simulink model "Test3S150Board_HSMA"  (Simulink 6.4)
settings: Solver=ode45  SolverMode=SingleTasking  StartTime=0.0  StopTime=1000.0  FixedStep=1  RelTol=1e-3
InitFcn:
  | %% DSPBuilder Start
  | alt_dspbuilder_update_model(bdroot)
  | %% DSPBuilder End
undefined symbols (not defined in the file): Pin_AA1, Pin_AA6, Pin_AA7, Pin_AB1, Pin_AB10, Pin_AB2, Pin_AB3, Pin_AB5, Pin_AB6, Pin_AB8, Pin_AC1, Pin_AC11, Pin_AC2, Pin_AC4, Pin_AC5, Pin_AC6, Pin_AC7, Pin_AC8, Pin_AC9, Pin_AD1, Pin_AD6, Pin_AD7, Pin_AE1, Pin_AE2, Pin_AE3, Pin_AE4, Pin_AE7, Pin_AE8, Pin_AF1, Pin_AF2, Pin_AF5, Pin_AF6, Pin_AG3, Pin_AG4, Pin_AH2, Pin_AH4, Pin_AH5, Pin_AJ1, Pin_AJ2, Pin_AJ3, Pin_AJ4, Pin_AJ9, Pin_AK1, Pin_AK9, Pin_AL1, Pin_AL2, Pin_AL7, Pin_AL9, Pin_AM1, Pin_AM2, Pin_Y10, Pin_Y5, Pin_Y6, Pin_Y7, Pin_Y8, Pin_Y9
libraries: allblocks_alteradspbuilder2 x49, Stratix_III_EP3SL150_alteradspbuilder2 x5
settings Model: Creator=lkong  LastModifiedBy=lkong
settings DataIOCC: SignalLoggingName=sigsOut
settings OptimizationCC: InlineInvariantSignals=on
settings DebuggingCC: SolverPrmCheckMsg=none  StrictBusMsg=None
settings HardwareCC: TargetUnknown=on
settings GRTTargetCC: ModelReferenceCompliant=off  MatFileLogging=off

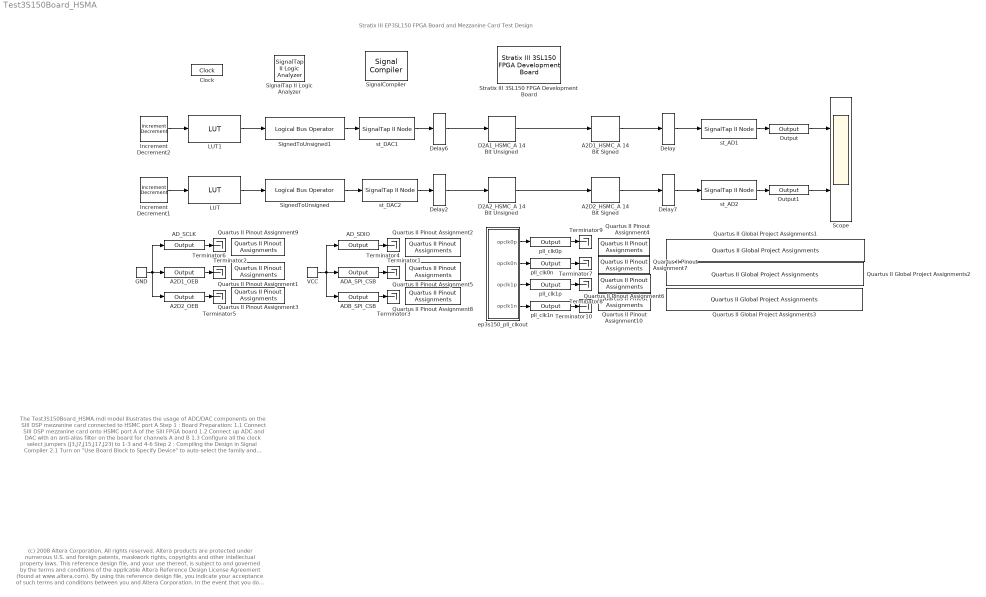
== system Test3S150Board_HSMA ==
  note: Stratix III EP3SL150 FPGA Board and Mezzanine Card Test Design
  note: (c) 2008 Altera Corporation. All rights reserved.  Altera products are protected under numerous U.S. and foreign patents, maskwork rights, copyrights and other intellectual property laws.
      | This reference design file, and your use thereof, is subject to and governed by the terms and conditions of the applicable Altera Reference Design License Agreement (found at www.altera.com).
      | By using this reference design file, you indicate your acceptance of such terms and conditions between you and Altera Corporation.
      | In the event that you do not agree with such terms and conditions, you may not use the reference design file and please promptly destroy any copies you have made.
      | This reference design file being provided on an "as-is" basis and as an accommodation and therefore all warranties, representations or guarantees of any kind (whether express, implied or statutory)
      | including, without limitation, warranties of merchantability, non-infringement, or fitness for a particular purpose, are specifically disclaimed.
      | By making this reference design file available, Altera expressly does not recommend, suggest or require that this reference design file be used in combination with any other product not provided by Altera
  note: The Test3S150Board_HSMA.mdl model illustrates the usage of ADC/DAC components on the SIII DSP mezzanine card connected to HSMC port A
      |
      | Step 1 : Board Preparation:
      |                1.1 Connect SIII DSP mezzanine card onto HSMC port A of the SIII FPGA board
      |                1.2 Connect up ADC and DAC with an anti-alias filter on the board for channels A and B
      |                1.3 Configure all the clock select jumpers (J3,J7,J15,J17,J23) to 1-3 and 4-6
      | Step 2 : Compiling the Design in Signal Compiler
      |                2.1 Turn on "Use Board Block to Specify Device" to auto-select the family and device
      |                2.2 Click "Compile" to compile the design through the Quartus II software and create a .sof file
      |                2.3 Click "Scan Jtag" to select a download cable and device
      |                2.4 Click "Program" to download the .sof file onto the FPGA device
      | Step 3 : Running SignalTap II Logic Analyzer
      |                3.1 Click "Scan Jtag" to select a download cable and device
      |                3.2 Click "Acquire" to obtain data for embedded SignalTap II nodes
  A2D1_HSMC_A 14 Bit Signed : Stratix_III_EP3SL150_alteradspbuilder2/A2D1_HSMC_A 14 Bit Signed  iofile=d:\ws80\workspace\Documentation\DesignExamples\Demos\Board\StratixIII_DSPBoard_3S150\tb_Test3S150Board_HSMA\Test3S150Board%5FHSMA_A2D1%5FHSMC%5FA+14+Bit+Signed.salt  externalType=Inferred  SpecifyClock=off  location=Pin_AD6,Pin_AD7,Pin_AF5,Pin_AF6,Pin_AE7,Pin_AE8,Pin_AH4,Pin_AH5,Pin_AC8,Pin_AC9,Pin_AB10,Pin_AC11,Pin_AL7,Pin_AK9
  A2D1_OEB : allblocks_alteradspbuilder2/Output  iofile=d:\ws80\workspace\Documentation\DesignExamples\Demos\Board\StratixIII_DSPBoard_3S150\tb_Test3S150Board_HSMA\Test3S150Board%5FHSMA_A2D1%5FOEB.capture  BusType=Single Bit  bwl=1  bwr=0  externalType=Inferred  PORTTYPE=Output  allowFloatingPointOverride=on  logOutputs=off
  A2D2_HSMC_A 14 Bit Signed : Stratix_III_EP3SL150_alteradspbuilder2/A2D2_HSMC_A 14 Bit Signed  iofile=d:\ws80\workspace\Documentation\DesignExamples\Demos\Board\StratixIII_DSPBoard_3S150\tb_Test3S150Board_HSMA\Test3S150Board%5FHSMA_A2D2%5FHSMC%5FA+14+Bit+Signed.salt  externalType=Inferred  SpecifyClock=off  location=Pin_AJ1,Pin_AH2,Pin_AK1,Pin_AJ2,Pin_AL1,Pin_AL2,Pin_AM1,Pin_AM2,Pin_AG3,Pin_AG4,Pin_AJ3,Pin_AJ4,Pin_AL9,Pin_AJ9
  A2D2_OEB : allblocks_alteradspbuilder2/Output  iofile=d:\ws80\workspace\Documentation\DesignExamples\Demos\Board\StratixIII_DSPBoard_3S150\tb_Test3S150Board_HSMA\Test3S150Board%5FHSMA_A2D2%5FOEB.capture  BusType=Single Bit  bwl=1  bwr=0  externalType=Inferred  PORTTYPE=Output  allowFloatingPointOverride=on  logOutputs=off
  ADA_SPI_CSB : allblocks_alteradspbuilder2/Output  iofile=d:\ws80\workspace\Documentation\DesignExamples\Demos\Board\StratixIII_DSPBoard_3S150\tb_Test3S150Board_HSMA\Test3S150Board%5FHSMA_ADA%5FSPI%5FCSB.capture  BusType=Single Bit  bwl=1  bwr=0  externalType=Inferred  PORTTYPE=Output  allowFloatingPointOverride=on  logOutputs=off
  ADB_SPI_CSB : allblocks_alteradspbuilder2/Output  iofile=d:\ws80\workspace\Documentation\DesignExamples\Demos\Board\StratixIII_DSPBoard_3S150\tb_Test3S150Board_HSMA\Test3S150Board%5FHSMA_ADB%5FSPI%5FCSB.capture  BusType=Single Bit  bwl=1  bwr=0  externalType=Inferred  PORTTYPE=Output  allowFloatingPointOverride=on  logOutputs=off
  AD_SCLK : allblocks_alteradspbuilder2/Output  iofile=d:\ws80\workspace\Documentation\DesignExamples\Demos\Board\StratixIII_DSPBoard_3S150\tb_Test3S150Board_HSMA\Test3S150Board%5FHSMA_AD%5FSCLK.capture  BusType=Single Bit  bwl=1  bwr=0  externalType=Inferred  PORTTYPE=Output  allowFloatingPointOverride=on  logOutputs=off
  AD_SDIO : allblocks_alteradspbuilder2/Output  iofile=d:\ws80\workspace\Documentation\DesignExamples\Demos\Board\StratixIII_DSPBoard_3S150\tb_Test3S150Board_HSMA\Test3S150Board%5FHSMA_AD%5FSDIO.capture  BusType=Single Bit  bwl=1  bwr=0  externalType=Inferred  PORTTYPE=Output  allowFloatingPointOverride=on  logOutputs=off
  Clock : allblocks_alteradspbuilder2/Clock  ClockPeriod=20  ClockPeriodUnit=ns  SampleTime=1  SimulationStartCycle=5  PhaseOffset=0  Reset=aclr  ResetType=Active Low  Export=off
  D2A1_HSMC_A 14 Bit Unsigned : Stratix_III_EP3SL150_alteradspbuilder2/D2A1_HSMC_A 14 Bit Unsigned  iofile=d:\ws80\workspace\Documentation\DesignExamples\Demos\Board\StratixIII_DSPBoard_3S150\tb_Test3S150Board_HSMA\Test3S150Board%5FHSMA_D2A1%5FHSMC%5FA+14+Bit+Unsigned.capture  externalType=Inferred  location=Pin_Y9,Pin_Y10,Pin_Y7,Pin_Y8,Pin_AA6,Pin_AA7,Pin_Y5,Pin_Y6,Pin_AC7,Pin_AB8,Pin_AB5,Pin_AB6,Pin_AC5,Pin_AC6
  D2A2_HSMC_A 14 Bit Unsigned : Stratix_III_EP3SL150_alteradspbuilder2/D2A2_HSMC_A 14 Bit Unsigned  iofile=d:\ws80\workspace\Documentation\DesignExamples\Demos\Board\StratixIII_DSPBoard_3S150\tb_Test3S150Board_HSMA\Test3S150Board%5FHSMA_D2A2%5FHSMC%5FA+14+Bit+Unsigned.capture  externalType=Inferred  location=Pin_AB3,Pin_AC4,Pin_AB1,Pin_AA1,Pin_AC1,Pin_AB2,Pin_AD1,Pin_AC2,Pin_AE3,Pin_AE4,Pin_AE1,Pin_AE2,Pin_AF1,Pin_AF2
  Delay : allblocks_alteradspbuilder2/Delay  pipeline=1  pipeline_display=1  ClockPhase=1  use_ena=off  use_sclr=off  allowFloatingPointOverride=on  logOutputs=off  logFile=d:\ws80\workspace\Documentation\DesignExamples\Demos\Board\StratixIII_DSPBoard_3S150\tb_Test3S150Board_HSMA\Test3S150Board%5FHSMA_Delay.fixedpointlog  use_init=off  reset_value=1
  Delay2 : allblocks_alteradspbuilder2/Delay  pipeline=1  pipeline_display=1  ClockPhase=1  use_ena=off  use_sclr=off  allowFloatingPointOverride=on  logOutputs=off  logFile=d:\ws80\workspace\Documentation\DesignExamples\Demos\Board\StratixIII_DSPBoard_3S150\tb_Test3S150Board_HSMA\Test3S150Board%5FHSMA_Delay2.fixedpointlog  use_init=off  reset_value=1
  Delay6 : allblocks_alteradspbuilder2/Delay  pipeline=1  pipeline_display=1  ClockPhase=1  use_ena=off  use_sclr=off  allowFloatingPointOverride=on  logOutputs=off  logFile=d:\ws80\workspace\Documentation\DesignExamples\Demos\Board\StratixIII_DSPBoard_3S150\tb_Test3S150Board_HSMA\Test3S150Board%5FHSMA_Delay6.fixedpointlog  use_init=off  reset_value=1
  Delay7 : allblocks_alteradspbuilder2/Delay  pipeline=1  pipeline_display=1  ClockPhase=1  use_ena=off  use_sclr=off  allowFloatingPointOverride=on  logOutputs=off  logFile=d:\ws80\workspace\Documentation\DesignExamples\Demos\Board\StratixIII_DSPBoard_3S150\tb_Test3S150Board_HSMA\Test3S150Board%5FHSMA_Delay7.fixedpointlog  use_init=off  reset_value=1
  GND : allblocks_alteradspbuilder2/GND  SpecifyClock=off
  Increment Decrement1 : allblocks_alteradspbuilder2/Increment Decrement  BusType=Unsigned Integer  bwl=7  bwr=0  SpecifyClock=off  clr_value=0  direction=Increment  phase_selection=1  use_ena=off  use_sclr=off  pipeline_display=1
  Increment Decrement2 : allblocks_alteradspbuilder2/Increment Decrement  BusType=Unsigned Integer  bwl=7  bwr=0  SpecifyClock=off  clr_value=0  direction=Increment  phase_selection=1  use_ena=off  use_sclr=off  pipeline_display=1
  LUT : allblocks_alteradspbuilder2/LUT  addr_width=7  BusType=Signed Integer  bwl=14  bwr=0  init_array=8191*sin( [0:2*pi/(2^7):2*pi] )  allowFloatingPointOverride=on  logOutputs=off  logFile=d:\ws80\workspace\Documentation\DesignExamples\Demos\Board\StratixIII_DSPBoard_3S150\tb_Test3S150Board_HSMA\Test3S150Board%5FHSMA_LUT.fixedpointlog  use_ena=off  reg_data=on  use_lpm=on  reg_addr=on  ram_type=AUTO  pipeline_display=2
  LUT1 : allblocks_alteradspbuilder2/LUT  addr_width=7  BusType=Signed Integer  bwl=14  bwr=0  init_array=8191*sin( [0:2*pi/(2^7):2*pi] )  allowFloatingPointOverride=on  logOutputs=off  logFile=d:\ws80\workspace\Documentation\DesignExamples\Demos\Board\StratixIII_DSPBoard_3S150\tb_Test3S150Board_HSMA\Test3S150Board%5FHSMA_LUT1.fixedpointlog  use_ena=off  reg_data=on  use_lpm=on  reg_addr=on  ram_type=AUTO  pipeline_display=2
  Output : allblocks_alteradspbuilder2/Output  iofile=d:\ws80\workspace\Documentation\DesignExamples\Demos\Board\StratixIII_DSPBoard_3S150\tb_Test3S150Board_HSMA\Test3S150Board%5FHSMA_Output.capture  BusType=Signed Integer  bwl=14  bwr=0  externalType=Inferred  PORTTYPE=Output  allowFloatingPointOverride=on  logOutputs=off
  Output1 : allblocks_alteradspbuilder2/Output  iofile=d:\ws80\workspace\Documentation\DesignExamples\Demos\Board\StratixIII_DSPBoard_3S150\tb_Test3S150Board_HSMA\Test3S150Board%5FHSMA_Output1.capture  BusType=Signed Integer  bwl=14  bwr=0  externalType=Inferred  PORTTYPE=Output  allowFloatingPointOverride=on  logOutputs=off
  Quartus II Global Project Assignments1 : allblocks_alteradspbuilder2/Quartus II Global Project Assignments  QuartusIIAssignmentName=RESERVE_DATA1_AFTER_CONFIGURATION  QuartusIIAssignmentValue="\"USE AS REGULAR IO\""
  Quartus II Global Project Assignments2 : allblocks_alteradspbuilder2/Quartus II Global Project Assignments  QuartusIIAssignmentName=RESERVE_NCEO_AFTER_CONFIGURATION  QuartusIIAssignmentValue="\"USE AS REGULAR IO\""
  Quartus II Global Project Assignments3 : allblocks_alteradspbuilder2/Quartus II Global Project Assignments  QuartusIIAssignmentName=RESERVE_DCLK_AFTER_CONFIGURATION  QuartusIIAssignmentValue="\"USE AS REGULAR IO\""
  Quartus II Pinout Assignment1 : allblocks_alteradspbuilder2/Quartus II Pinout Assignments  QuartusIIAssignmentName=A2D1_OEB  QuartusIIAssignmentValue=Pin_AE5
  Quartus II Pinout Assignment10 : allblocks_alteradspbuilder2/Quartus II Pinout Assignments  QuartusIIAssignmentName=pll_clk1n  QuartusIIAssignmentValue=Pin_W7
  Quartus II Pinout Assignment2 : allblocks_alteradspbuilder2/Quartus II Pinout Assignments  QuartusIIAssignmentName=AD_SDIO  QuartusIIAssignmentValue=Pin_AD3
  Quartus II Pinout Assignment3 : allblocks_alteradspbuilder2/Quartus II Pinout Assignments  QuartusIIAssignmentName=A2D2_OEB  QuartusIIAssignmentValue=Pin_AF3
  Quartus II Pinout Assignment4 : allblocks_alteradspbuilder2/Quartus II Pinout Assignments  QuartusIIAssignmentName=pll_clk0p  QuartusIIAssignmentValue=Pin_V10
  Quartus II Pinout Assignment5 : allblocks_alteradspbuilder2/Quartus II Pinout Assignments  QuartusIIAssignmentName=ADA_SPI_CSB  QuartusIIAssignmentValue=Pin_AD4
  Quartus II Pinout Assignment6 : allblocks_alteradspbuilder2/Quartus II Pinout Assignments  QuartusIIAssignmentName=pll_clk1p  QuartusIIAssignmentValue=Pin_W8
  Quartus II Pinout Assignment7 : allblocks_alteradspbuilder2/Quartus II Pinout Assignments  QuartusIIAssignmentName=pll_clk0n  QuartusIIAssignmentValue=Pin_W9
  Quartus II Pinout Assignment8 : allblocks_alteradspbuilder2/Quartus II Pinout Assignments  QuartusIIAssignmentName=ADB_SPI_CSB  QuartusIIAssignmentValue=Pin_AG1
  Quartus II Pinout Assignment9 : allblocks_alteradspbuilder2/Quartus II Pinout Assignments  QuartusIIAssignmentName=AD_SCLK  QuartusIIAssignmentValue=Pin_AH1
  Scope : Scope  NumInputPorts=2
      settings: YMin=-5~-5  YMax=5~5  SampleInput=on
  SignalCompiler : allblocks_alteradspbuilder2/Signal Compiler  DeviceFamily=Stratix III  DeviceName=EP3SL150F1152C4  EnableSignalTap=on  SignalTapDepth=512  UseBoardBlock=on  StpUseDefaultClock=on  StpClock=Clock  ExportDir=D:\MATLAB\R2006a\work
  SignalTap II Logic Analyzer : allblocks_alteradspbuilder2/SignalTap II Logic Analyzer
  SignedToUnsigned : allblocks_alteradspbuilder2/Logical Bus Operator  BusType=Unsigned Integer  bwl=14  bwr=0  LogicalOp_text=XOR  mask_value_num=8192  shift_amount=3  force_sign_ext=off  pipeline_display=0
  SignedToUnsigned1 : allblocks_alteradspbuilder2/Logical Bus Operator  BusType=Unsigned Integer  bwl=14  bwr=0  LogicalOp_text=XOR  mask_value_num=8192  shift_amount=3  force_sign_ext=off  pipeline_display=0
  "Stratix III 3SL150 FPGA Development Board " : Stratix_III_EP3SL150_alteradspbuilder2/Stratix III 3SL150 FPGA Development Board   ClockPinIn=Pin_T33  GlobalResetPin=PIN_AP5  device=EP3SL150F1152C4
  Terminator{1..10} (10 alike) : Terminator
  VCC : allblocks_alteradspbuilder2/VCC  SpecifyClock=off
  ep3s150_pll_clkout : Subsystem
      mask Type: SubSystem AlteraBlockSet
  pll_clk0n : allblocks_alteradspbuilder2/Output  iofile=d:\ws80\workspace\Documentation\DesignExamples\Demos\Board\StratixIII_DSPBoard_3S150\tb_Test3S150Board_HSMA\Test3S150Board%5FHSMA_pll%5Fclk0n.capture  BusType=Single Bit  bwl=1  bwr=0  externalType=Inferred  PORTTYPE=Output  allowFloatingPointOverride=on  logOutputs=off
  pll_clk0p : allblocks_alteradspbuilder2/Output  iofile=d:\ws80\workspace\Documentation\DesignExamples\Demos\Board\StratixIII_DSPBoard_3S150\tb_Test3S150Board_HSMA\Test3S150Board%5FHSMA_pll%5Fclk0p.capture  BusType=Single Bit  bwl=1  bwr=0  externalType=Inferred  PORTTYPE=Output  allowFloatingPointOverride=on  logOutputs=off
  pll_clk1n : allblocks_alteradspbuilder2/Output  iofile=d:\ws80\workspace\Documentation\DesignExamples\Demos\Board\StratixIII_DSPBoard_3S150\tb_Test3S150Board_HSMA\Test3S150Board%5FHSMA_pll%5Fclk1n.capture  BusType=Single Bit  bwl=1  bwr=0  externalType=Inferred  PORTTYPE=Output  allowFloatingPointOverride=on  logOutputs=off
  pll_clk1p : allblocks_alteradspbuilder2/Output  iofile=d:\ws80\workspace\Documentation\DesignExamples\Demos\Board\StratixIII_DSPBoard_3S150\tb_Test3S150Board_HSMA\Test3S150Board%5FHSMA_pll%5Fclk1p.capture  BusType=Single Bit  bwl=1  bwr=0  externalType=Inferred  PORTTYPE=Output  allowFloatingPointOverride=on  logOutputs=off
  st_AD1 : allblocks_alteradspbuilder2/SignalTap II Node  id=0
  st_AD2 : allblocks_alteradspbuilder2/SignalTap II Node  id=1
  st_DAC1 : allblocks_alteradspbuilder2/SignalTap II Node  id=2
  st_DAC2 : allblocks_alteradspbuilder2/SignalTap II Node  id=3
  wires:
  SignedToUnsigned1/1 -> st_DAC1/1
  Delay/1 -> st_AD1/1
  Delay6/1 -> D2A1_HSMC_A 14 Bit Unsigned/1
  st_DAC1/1 -> Delay6/1
  D2A1_HSMC_A 14 Bit Unsigned/1 -> A2D1_HSMC_A 14 Bit Signed/1
  LUT/1 -> SignedToUnsigned/1
  SignedToUnsigned/1 -> st_DAC2/1
  Increment Decrement1/1 -> LUT/1
  Delay2/1 -> D2A2_HSMC_A 14 Bit Unsigned/1
  st_DAC2/1 -> Delay2/1
  D2A2_HSMC_A 14 Bit Unsigned/1 -> A2D2_HSMC_A 14 Bit Signed/1
  A2D1_HSMC_A 14 Bit Signed/1 -> Delay/1
  A2D2_HSMC_A 14 Bit Signed/1 -> Delay7/1
  Delay7/1 -> st_AD2/1
  st_AD1/1 -> Output/1
  st_AD2/1 -> Output1/1
  Output/1 -> Scope/1
  Output1/1 -> Scope/2
  LUT1/1 -> SignedToUnsigned1/1
  Increment Decrement2/1 -> LUT1/1
  A2D1_OEB/1 -> Terminator2/1
  A2D2_OEB/1 -> Terminator5/1
  ADA_SPI_CSB/1 -> Terminator1/1
  ADB_SPI_CSB/1 -> Terminator3/1
  VCC/1 -> ADB_SPI_CSB/1, ADA_SPI_CSB/1, AD_SDIO/1
  AD_SDIO/1 -> Terminator4/1
  AD_SCLK/1 -> Terminator6/1
  ep3s150_pll_clkout/1(opclk0p) -> pll_clk0p/1
  ep3s150_pll_clkout/2(opclk0n) -> pll_clk0n/1
  ep3s150_pll_clkout/3(opclk1p) -> pll_clk1p/1
  ep3s150_pll_clkout/4(opclk1n) -> pll_clk1n/1
  pll_clk0p/1 -> Terminator9/1
  pll_clk0n/1 -> Terminator7/1
  pll_clk1p/1 -> Terminator8/1
  pll_clk1n/1 -> Terminator10/1
  GND/1 -> A2D2_OEB/1, AD_SCLK/1, A2D1_OEB/1

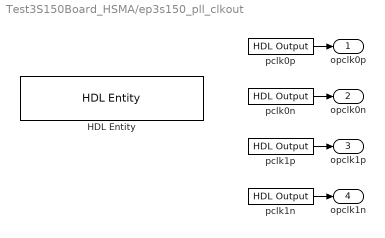
== system Test3S150Board_HSMA/ep3s150_pll_clkout ==
  HDL Entity : allblocks_alteradspbuilder2/HDL Entity  HDLFile=ep3s150_pll_clkout.vhd  clockname=clkin_50  useSubsystemPortName=off
  pclk0n : allblocks_alteradspbuilder2/HDL Output  BusType=Single Bit  bwl=1  bwr=0  externalType=Inferred
  pclk0p : allblocks_alteradspbuilder2/HDL Output  BusType=Single Bit  bwl=1  bwr=0  externalType=Inferred
  pclk1n : allblocks_alteradspbuilder2/HDL Output  BusType=Single Bit  bwl=1  bwr=0  externalType=Inferred
  pclk1p : allblocks_alteradspbuilder2/HDL Output  BusType=Single Bit  bwl=1  bwr=0  externalType=Inferred
  opclk0p : Outport
  opclk0n : Outport  Port=2
  opclk1p : Outport  Port=3
  opclk1n : Outport  Port=4
  wires:
  pclk0p/1 -> opclk0p/1
  pclk0n/1 -> opclk0n/1
  pclk1p/1 -> opclk1p/1
  pclk1n/1 -> opclk1n/1
